simulink model "VIRTUAL_self_driving_stack_v2"  (R2024a)
settings: Solver=ode1  StartTime=0.0  StopTime=inf  FixedStep=Controller_Sample_Time  RelTol=1e-3  EnableMultiTasking=on
values from neighbouring files (symbols this model uses):
  angles_qcar2 = angles_new_qcar2(2: length (angles_new_qcar2), width (angles_new_qcar2)-5)    [Setup_QCar2_Params.m]
  cal_pos = [0, 0, 0]    [Setup_QCar2_Params.m]    (also in Setup_QCar2_Params_Addons.m)
  Controller_Sample_Time = 1/500    (= 0.002)    [Setup_QCar2_Params.m]    (also in Setup_QCar2_Params_Addons.m)
  CSI_Sample_Time = Controller_Sample_Time * ceil(0.033 / Controller_Sample_Time)    [Setup_QCar2_Params.m]
  GyroKF_P0 = eye(2)    [Setup_QCar2_Params.m]
  GyroKF_Q = diag([0.01, 0.001])    [Setup_QCar2_Params.m]
  GyroKF_R = 0.01    [Setup_QCar2_Params.m]
  GyroKF_X0 = [0;0]    [Setup_QCar2_Params.m]
  ImageDisplay_Sample_Time = Controller_Sample_Time * 50    (= 0.1)    [Setup_QCar2_Params.m]
  Initialization_Time = 5    [Setup_QCar2_Params.m]
  LiDAR_Sample_Time = Controller_Sample_Time * ceil(1/15 / Controller_Sample_Time)    [Setup_QCar2_Params.m]
  qcar2_lidar_to_body_rotation = -pi    (= -3.14159265359)    [Setup_QCar2_Params.m]
  qcar2_lidar_to_map_rotation = 0    [Setup_QCar2_Params.m]
  qcar2_virtual_to_physical_lidar_rotation = 0    [Setup_QCar2_Params.m]
  QCarEKF_L = 0.256    [Setup_QCar2_Params.m]
  QCarEKF_P0 = eye(3)    [Setup_QCar2_Params.m]
  QCarEKF_Q = diag([0.00001, 0.00001, 0.00001])    [Setup_QCar2_Params.m]
  QCarEKF_R_combined = diag([0.1, 0.1, 0.01])    [Setup_QCar2_Params.m]
  QCarEKF_R_heading = diag(0.1)    [Setup_QCar2_Params.m]
  QcarKF_X0 = [0; 0; 0]    [Setup_QCar2_Params.m]
  range_qcar2 = distance_new_qcar2(2: length (distance_new_qcar2), width (distance_new_qcar2)-5)    [Setup_QCar2_Params.m]
  RealSense_Sample_Time = Controller_Sample_Time * ceil(0.033 / Controller_Sample_Time)    [Setup_QCar2_Params.m]
undefined symbols (not defined in the file or in its folder): AAAF5050, gcbh, height, HIL, JPEG, K12, left, MC, path_x4, path_y4, Point, qc_get_step_size, top, video_display_show, width
libraries: quarc_library x42, simulink x3, simulink_extras x3
(part 1 of 2)
settings Model: SimulationMode=external  ExtModeTrigDuration=10000  Creator=PKaram  LastModifiedBy=mgilewicz
settings SolverCC: AlgebraicLoopSolver=TrustRegion  PositivePriorityOrder=on  AutoInsertRateTranBlk=on
settings DataIOCC: ReturnWorkspaceOutputs=off
settings DebuggingCC: ParameterPrecisionLossMsg=none  UnconnectedInputMsg=warning  UnconnectedOutputMsg=warning  UnconnectedLineMsg=warning  ArithmeticOperatorsInVariantConditions=warning
settings ModelReferenceCC: EnableRefExpFcnMdlSchedulingChecks=on
settings SFSimCC: SimUseLocalCustomCode=off  CustomCodeUndefinedFunction=UseInterfaceOnly
settings RTWCC: Description=QUARC Win64 Target Using Toolchain  SystemTargetFile=quarc_win64.tlc  TemplateMakefile=quarc_linux_nvidia_tmf  RTWUseLocalCustomCode=off  Toolchain=QUARC win64 | nmake (64-bit Windows)  BuildConfiguration=Faster Runs  GPUComputeCapability=3.5  DLArmComputeVersion=19.05
settings CodeAppCC: StateflowObjectComments=on
settings STFCustomTargetCC: ConcurrentExecutionCompliant=on  SystemTargetFile=quarc_win64.tlc
settings GRTTargetCC: ParMdlRefBuildCompliant=off  CompOptLevelCompliant=off  CombineOutputUpdateFcns=off  MatFileLogging=off  CPPClassGenCompliant=off  GRTInterface=on  ExtMode=on  ExtModeMexFile=quarc_comm
settings ConfigComp: CovMetricSettings=dswe  CovBoundaryAbsTol=1.0e-5

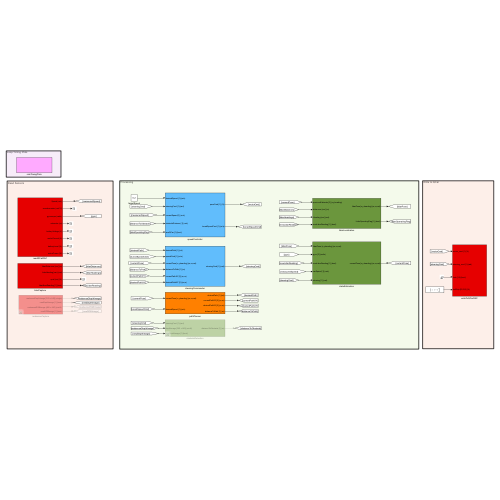
[thumbnail: Simulink's stored preview of the top-level diagram]
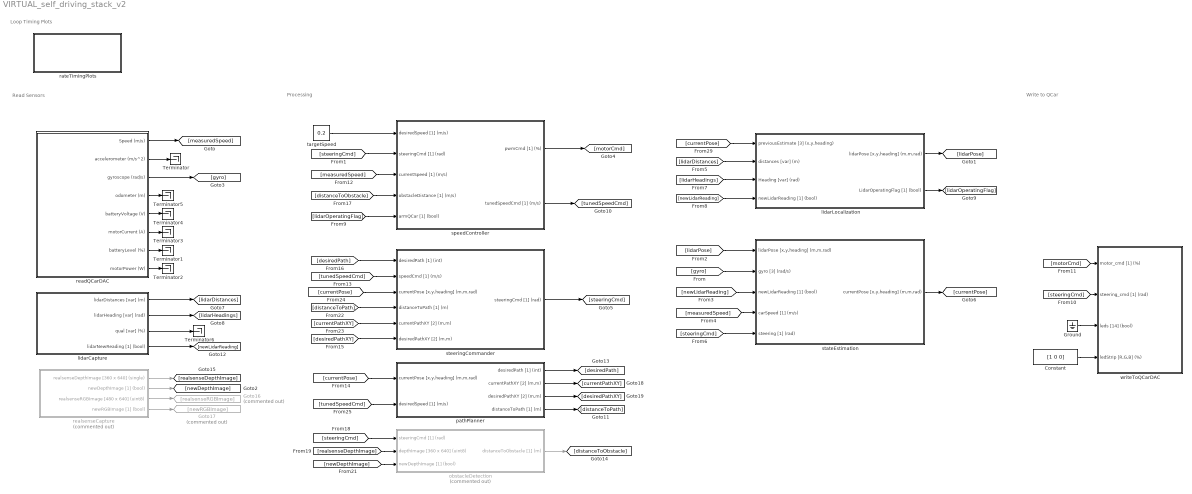
== system VIRTUAL_self_driving_stack_v2 ==
  note: Loop Timing Plots
  note: Write to QCar
  note: Processing
  note: Read Sensors
  Constant : Constant  Value=[1 0 0]
  Goto16 : Goto  Commented=on  GotoTag=realsenseRGBImage
  Goto17 : Goto  Commented=on  GotoTag=newRGBImage
  Ground : Ground
  Terminator{,1..6} (7 alike) : Terminator
  lidarCapture : Subsystem
  lidarLocalization : Subsystem
  obstacleDetection : Subsystem  Commented=on
  pathPlanner : Subsystem
  rateTimingPlots : Subsystem
  readQCarDAC : Subsystem
  realsenseCapture : Subsystem  Commented=on
  speedController : Subsystem
  stateEstimation : Subsystem
  steeringCommander : Subsystem
  targetSpeed : Constant  Value=0.2
  writeToQCarDAC : Subsystem
  wires:
  readQCarDAC/6(motorCurrent (A)) -> Terminator3/1
  [measuredSpeed] -> stateEstimation/4(carSpeed [1] (m/s))
  [newLidarReading] -> stateEstimation/3(newLidarReading [1] (bool))
  [tunedSpeedCmd] -> steeringCommander/2(speedCmd [1] (m/s))
  Constant/1 -> writeToQCarDAC/4(ledStrip [R,G,B] (%))
  pathPlanner/2(currentPathXY [2] (m,m)) -> [currentPathXY]
  lidarCapture/2(lidarHeading [var] (rad)) -> [lidarHeadings]
  readQCarDAC/2(accelerometer (m/s^2)) -> Terminator/1
  lidarLocalization/2(LidarOperatingFlag [1] (bool)) -> [lidarOperatingFlag]
  Ground/1 -> writeToQCarDAC/3(leds [14] (bool))
  [lidarHeadings] -> lidarLocalization/3(Heading [var] (rad))
  realsenseCapture/1(realsenseDepthImage [360 x 640] (single)) -> [realsenseDepthImage]
  [steeringCmd] -> writeToQCarDAC/2(steering_cmd [1] (rad))
  pathPlanner/4(distanceToPath [1] (m)) -> [distanceToPath]
  lidarCapture/1(lidarDistances [var] (m)) -> [lidarDistances]
  readQCarDAC/4(odometer (m)) -> Terminator5/1
  readQCarDAC/3(gyroscope (rad/s)) -> [gyro]
  pathPlanner/3(desiredPathXY [2] (m,m)) -> [desiredPathXY]
  [newLidarReading] -> lidarLocalization/4(newLidarReading [1] (bool))
  [newDepthImage] -> obstacleDetection/3(newDepthImage [1] (bool))
  [tunedSpeedCmd] -> pathPlanner/2(desiredSpeed [1] (m/s))
  readQCarDAC/5(batteryVoltage (V)) -> Terminator4/1
  readQCarDAC/1(Speed (m/s)) -> [measuredSpeed]
  speedController/2(tunedSpeedCmd [1] (m/s)) -> [tunedSpeedCmd]
  [distanceToObstacle] -> speedController/4(obstacleDistance [1] (m/s))
  [gyro] -> stateEstimation/2(gyro [3] (rad/s))
  [currentPathXY] -> steeringCommander/5(currentPathXY [2] (m,m))
  [lidarPose] -> stateEstimation/1(lidarPose [x,y,heading] (m,m,rad))
  targetSpeed/1 -> speedController/1(desiredSpeed [1] (m/s))
  [steeringCmd] -> stateEstimation/5(steering [1] (rad))
  [realsenseDepthImage] -> obstacleDetection/2(depthImage [360 x 640] (uint8))
  readQCarDAC/8(motorPower (W)) -> Terminator2/1
  speedController/1(pwmCmd [1] (%)) -> [motorCmd]
  [lidarDistances] -> lidarLocalization/2(distances [var] (m))
  [lidarOperatingFlag] -> speedController/5(armQCar [1] (bool))
  [motorCmd] -> writeToQCarDAC/1(motor_cmd [1] (%))
  [steeringCmd] -> speedController/2(steeringCmd [1] (rad))
  lidarCapture/4(lidarNewReading [1] (bool)) -> [newLidarReading]
  lidarLocalization/1(lidarPose [x,y,heading] (m,m,rad)) -> [lidarPose]
  [desiredPathXY] -> steeringCommander/6(desiredPathXY [2] (m,m))
  [distanceToPath] -> steeringCommander/4(distanceToPath [1] (m))
  realsenseCapture/4(newRGBImage [1] (bool)) -> Goto17/1
  lidarCapture/3(qual [var] (%)) -> Terminator6/1
  readQCarDAC/7(batteryLevel (%)) -> Terminator1/1
  [desiredPath] -> steeringCommander/1(desiredPath [1] (int))
  [steeringCmd] -> obstacleDetection/1(steeringCmd [1] (rad))
  steeringCommander/1(steeringCmd [1] (rad)) -> [steeringCmd]
  obstacleDetection/1(distanceToObstacle [1] (m)) -> [distanceToObstacle]
  [measuredSpeed] -> speedController/3(currentSpeed [1] (m/s))
  pathPlanner/1(desiredPath [1] (int)) -> [desiredPath]
  realsenseCapture/2(newDepthImage [1] (bool)) -> [newDepthImage]
  realsenseCapture/3("realsenseRGBImage [480 x 640] (uint8) ") -> Goto16/1
  stateEstimation/1(currentPose [x,y,heading] (m,m,rad)) -> [currentPose]
  [currentPose] -> pathPlanner/1(currentPose [x,y,heading] (m,m,rad))
  [currentPose] -> steeringCommander/3(currentPose [x,y,heading] (m,m,rad))
  [currentPose] -> lidarLocalization/1(previousEstimate [3] (x,y,heading))

== system VIRTUAL_self_driving_stack_v2/lidarCapture ==
  Ranging Sensor : quarc_library/Devices/Third-Party/Sensors/Ranging Sensor  sensor_type=RPLidar LIDAR  uri=tcpip://localhost:18966  ranging_distance=Long  timing_budget=0.033  measurement_period=0.040  output_mode=Variable-size output  samples_per_revolution=SPR_qcar2  max_distance=0.050  max_angle=5  sample_time=LiDAR_Sample_Time  show_versions=on  active=on
      settings: SourceProductName=QUARC Targets
  Terminator : Terminator
  lidarFirmwareVer : Display
      settings: Decimation=100
  lidarHardwareVer : Display
      settings: Decimation=100
  lidarModel : Display
      settings: Decimation=100
  virtualLidarToPhysicalLidarOffset : Bias  Bias=qcar2_virtual_to_physical_lidar_rotation  SaturateOnIntegerOverflow=off
  lidarDistances [var] (m) : Outport  VectorParamsAs1DForOutWhenUnconnected=off
  lidarHeading [var] (rad) : Outport  Port=2  VectorParamsAs1DForOutWhenUnconnected=off
  qual [var] (%) : Outport  Port=3  VectorParamsAs1DForOutWhenUnconnected=off
  lidarNewReading [1] (bool) : Outport  Port=4  VectorParamsAs1DForOutWhenUnconnected=off
  wires:
  Ranging Sensor/3 -> virtualLidarToPhysicalLidarOffset/1
  Ranging Sensor/5 -> lidarNewReading [1] (bool)/1
  Ranging Sensor/7 -> lidarHardwareVer/1
  Ranging Sensor/8 -> lidarFirmwareVer/1
  Ranging Sensor/6 -> lidarModel/1
  Ranging Sensor/4 -> qual [var] (%)/1
  Ranging Sensor/1 -> lidarDistances [var] (m)/1
  Ranging Sensor/2 -> Terminator/1
  virtualLidarToPhysicalLidarOffset/1 -> lidarHeading [var] (rad)/1

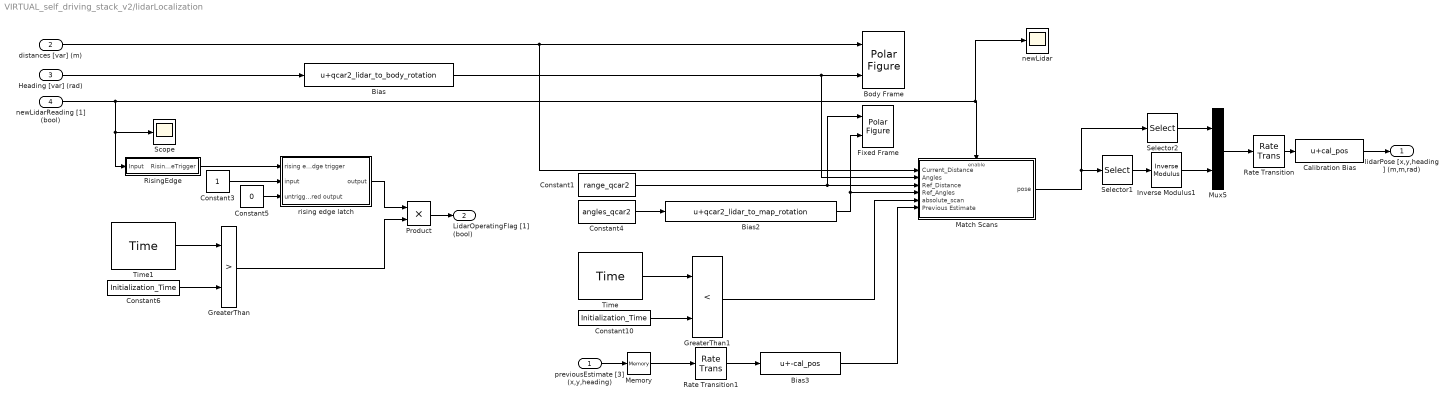
== system VIRTUAL_self_driving_stack_v2/lidarLocalization ==
  previousEstimate [3] (x,y,heading) : Inport
  distances [var] (m) : Inport  Port=2
  Heading [var] (rad) : Inport  Port=3
  newLidarReading [1] (bool) : Inport  Port=4
  Bias : Bias  Bias=qcar2_lidar_to_body_rotation  SaturateOnIntegerOverflow=off
  Bias2 : Bias  Bias=qcar2_lidar_to_map_rotation  SaturateOnIntegerOverflow=off
  Bias3 : Bias  Bias=-cal_pos  SaturateOnIntegerOverflow=off
  Body Frame : quarc_library/Sinks/Figures/Polar Figure  figure_mode=Use figure window  figure_tag=figure1  axes_tag=axes1  plot_mode=Frame-based  minimum_rho=0  maximum_rho=10  minimum_theta=0  maximum_theta=360  zero_location=top  direction=clockwise  buffer_size=SPR_qcar2  update_rate=1  sample_time=-1  initial_position="-958   50  958  973"  initial_visibility=off  line1_style=None  line1_width=0.5  line1_color=[0 0.4470 0.7410]  marker1=Point (.)  marker1_size=1  marker1_edge_color=[0 0.447059 0.741176]  marker1_face_color=[0 0.447059 0.741176]  line2_style=Solid line (-)  line2_width=0.5  line2_color=[0.85098 0.32549 0.0980392]  marker2=None  marker2_size=6  marker2_edge_color=[0.85098 0.32549 0.0980392]  marker2_face_color=[0.85098 0.32549 0.0980392]  line3_style=Solid line (-)  line3_width=0.5  line3_color=[0.929412 0.694118 0.12549]  marker3=None  marker3_size=6  marker3_edge_color=[0.929412 0.694118 0.12549]  marker3_face_color=[0.929412 0.694118 0.12549]  line4_style=Solid line (-)  line4_width=0.5  line4_color=[0.494118 0.184314 0.556863]  marker4=None  marker4_size=6  marker4_edge_color=[0.494118 0.184314 0.556863]  marker4_face_color=[0.494118 0.184314 0.556863]  line5_style=Solid line (-)  line5_width=0.5  line5_color=[0.466667 0.67451 0.188235]  marker5=None  marker5_size=6  marker5_edge_color=[0.466667 0.67451 0.188235]  marker5_face_color=[0.466667 0.67451 0.188235]
      settings: SourceProductName=QUARC Targets
  Calibration Bias : Bias  Bias=cal_pos  SaturateOnIntegerOverflow=off
  Constant1 : Constant  Value=range_qcar2
  Constant10 : Constant  Value=Initialization_Time
  Constant3 : Constant
  Constant4 : Constant  Value=angles_qcar2
  Constant5 : Constant  Value=0
  Constant6 : Constant  Value=Initialization_Time
  Fixed Frame : quarc_library/Sinks/Figures/Polar Figure  figure_mode=Use figure window  figure_tag=figure1  axes_tag=axes1  plot_mode=Frame-based  minimum_rho=0  maximum_rho=6  minimum_theta=0  maximum_theta=360  zero_location=top  direction=clockwise  buffer_size=SPR_qcar2  update_rate=1  sample_time=-1  initial_position="-1918    50   958   973"  initial_visibility=off  line1_style=None  line1_width=0.5  line1_color=[0 0.4470 0.7410]  marker1=Point (.)  marker1_size=1  marker1_edge_color=[0 0.447059 0.741176]  marker1_face_color=[0 0.447059 0.741176]  line2_style=Solid line (-)  line2_width=0.5  line2_color=[0.85098 0.32549 0.0980392]  marker2=None  marker2_size=6  marker2_edge_color=[0.85098 0.32549 0.0980392]  marker2_face_color=[0.85098 0.32549 0.0980392]  line3_style=Solid line (-)  line3_width=0.5  line3_color=[0.929412 0.694118 0.12549]  marker3=None  marker3_size=6  marker3_edge_color=[0.929412 0.694118 0.12549]  marker3_face_color=[0.929412 0.694118 0.12549]  line4_style=Solid line (-)  line4_width=0.5  line4_color=[0.494118 0.184314 0.556863]  marker4=None  marker4_size=6  marker4_edge_color=[0.494118 0.184314 0.556863]  marker4_face_color=[0.494118 0.184314 0.556863]  line5_style=Solid line (-)  line5_width=0.5  line5_color=[0.466667 0.67451 0.188235]  marker5=None  marker5_size=6  marker5_edge_color=[0.466667 0.67451 0.188235]  marker5_face_color=[0.466667 0.67451 0.188235]
      settings: SourceProductName=QUARC Targets
  GreaterThan : RelationalOperator  Operator=>  OutDataTypeStr=boolean  RndMeth=Simplest  InputSameDT=off
  GreaterThan1 : RelationalOperator  Operator=<  OutDataTypeStr=boolean  RndMeth=Simplest  InputSameDT=off
  Inverse Modulus1 : quarc_library/Discontinuities/Inverse Modulus  modulus=2*pi  output_derivative=off  output_revolutions=off  max_x=Inf  min_x=-Inf
  Match Scans : Subsystem
  Memory : Memory
  Mux5 : Mux  Inputs=2
  Product : Product
  Rate Transition : RateTransition
  Rate Transition1 : RateTransition
  RisingEdge : Subsystem
  Scope : Scope
  Selector1 : Selector  InputPortWidth=3  IndexOptions=Index vector (dialog)  Indices=3  OutputSizes=1
  Selector2 : Selector  InputPortWidth=3  IndexOptions=Index vector (dialog)  Indices=1:2  OutputSizes=1
  Time : quarc_library/Sources/Time/Time  time_source=Wall clock  sample_time=LiDAR_Sample_Time
  Time1 : quarc_library/Sources/Time/Time  time_source=Wall clock  sample_time=qc_get_step_size
  newLidar : Scope
  rising edge latch : Subsystem
  lidarPose [x,y,heading] (m,m,rad) : Outport
  LidarOperatingFlag [1] (bool) : Outport  Port=2
  wires:
  RisingEdge/1(RisingEdgeTrigger) -> rising edge latch/1(rising edge trigger)
  Bias3/1 -> Match Scans/6(Previous Estimate)
  Inverse Modulus1/1 -> Mux5/2
  Constant1/1 -> Fixed Frame/1, Match Scans/3(Ref_Distance)
  Time1/1 -> GreaterThan/1
  Rate Transition1/1 -> Bias3/1
  Bias2/1 -> Fixed Frame/2, Match Scans/4(Ref_Angles)
  Constant3/1 -> rising edge latch/2(input)
  GreaterThan/1 -> Product/2
  Selector2/1 -> Mux5/1
  Bias/1 -> Body Frame/2, Match Scans/2(Angles)
  Constant10/1 -> GreaterThan1/2
  Mux5/1 -> Rate Transition/1
  rising edge latch/1(output) -> Product/1
  Constant6/1 -> GreaterThan/2
  Heading [var] (rad)/1 -> Bias/1
  distances [var] (m)/1 -> Match Scans/1(Current_Distance), Body Frame/1
  Time/1 -> GreaterThan1/1
  Match Scans/1(pose) -> Selector2/1, Selector1/1
  Product/1 -> LidarOperatingFlag [1] (bool)/1
  Constant4/1 -> Bias2/1
  newLidarReading [1] (bool)/1 -> newLidar/1, Match Scans/Enable, RisingEdge/1(Input), Scope/1
  GreaterThan1/1 -> Match Scans/5(absolute_scan)
  Selector1/1 -> Inverse Modulus1/1
  Calibration Bias/1 -> lidarPose [x,y,heading] (m,m,rad)/1
  previousEstimate [3] (x,y,heading)/1 -> Memory/1
  Rate Transition/1 -> Calibration Bias/1
  Constant5/1 -> rising edge latch/3(untriggered output)
  Memory/1 -> Rate Transition1/1

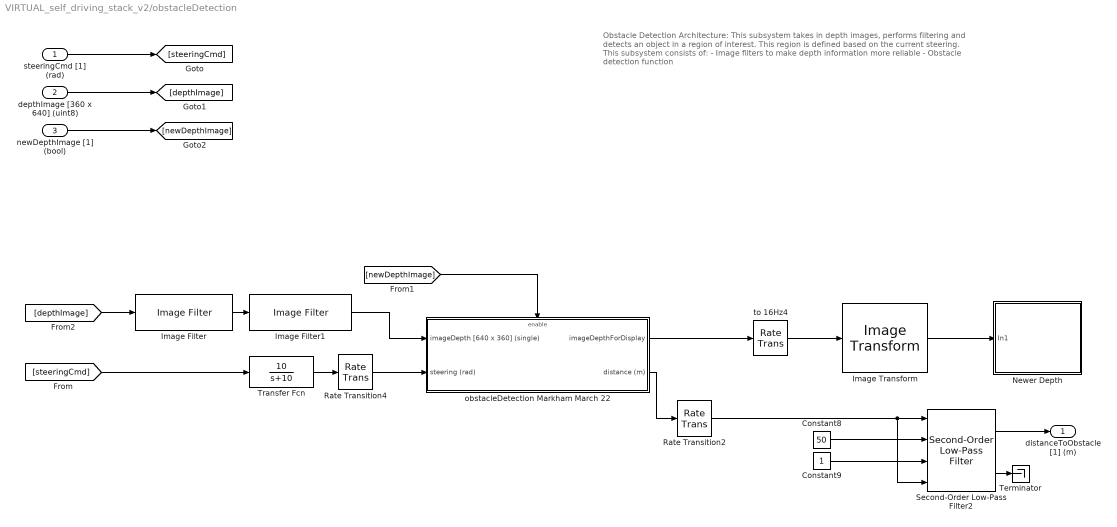
== system VIRTUAL_self_driving_stack_v2/obstacleDetection ==
  note: Obstacle Detection Architecture:
      |
      | This subsystem takes in depth images, performs filtering and detects an object in a region of interest. This region is defined based on the current steering.
      |
      | This subsystem consists of:
      |
      | - Image filters to make depth information more reliable
      | - Obstacle detection function
  steeringCmd [1] (rad) : Inport
  depthImage [360 x 640] (uint8) : Inport  Port=2
  newDepthImage [1] (bool) : Inport  Port=3
  Constant8 : Constant  Value=50
  Constant9 : Constant
  Image Filter : quarc_library/Image Processing/Generic/Image Filter  filter_type=Depth hole-fill  source_of_roi=Internal dialog parameter  roi_style=[top, left, height, width]  roi=[]  maximum_roi=[]  roi_zone=Operate inside region of interest  border_type=Replicate  border_value=[0 0 0]  kernel_size=5  sigma=10  mask_size=[3 3]  kernel=int16([-2 -1 0; -1 1 1; 0 1 2])  divisor=1  offset=0  rounding=Nearest  algorithm_hint=None  threshold=100  alpha=0.9  num_frames=8  num_valid=1  gap_threshold=10  depth_threshold=255  iterations=2  norm_type=L1
      settings: AttributesFormatString=(%<filter_type>)  SourceProductName=QUARC Targets
  Image Filter1 : quarc_library/Image Processing/Generic/Image Filter  filter_type=Depth temporal low-pass  source_of_roi=Internal dialog parameter  roi_style=[top, left, height, width]  roi=[]  maximum_roi=[]  roi_zone=Operate inside region of interest  border_type=Replicate  border_value=[0 0 0]  kernel_size=5  sigma=10  mask_size=[3 3]  kernel=int16([-2 -1 0; -1 1 1; 0 1 2])  divisor=1  offset=0  rounding=Nearest  algorithm_hint=None  threshold=100  alpha=0.9  num_frames=4  num_valid=1  gap_threshold=10  depth_threshold=255  iterations=2  norm_type=L1
      settings: AttributesFormatString=(%<filter_type>)  SourceProductName=QUARC Targets
  Image Transform : quarc_library/Image Processing/Generic/Image Transform  algorithm=Colorize  color_theme=KRYGCBMW  min_pixel=0  max_pixel=65535  contour_depth=1  focal_length=308  principal_point=[262 334]  radial_coeffs=[-0.3129 0.0907]  tangential_coeffs=[]  extrapolated_pixel=0  interpolation=nearest  row_coords=0  column_coords=0  output_height=480  output_width=640  angle=0  origin=[240 320]  output_origin=[240 320]  output_data_type=uint8
      settings: AttributesFormatString=(%<algorithm>)  SourceProductName=QUARC Targets
  Newer Depth : Subsystem  LoadFcn=set_param(gcbh, 'UserData', gcb);  StartFcn=video_display_show([gcb, '/Video Display'], 'add', gcb);  mask(Video Compressed Display){algorithm=JPEG, quality=50, sample_time=-1, use_hardware=on}
      mask prompts: algorithm "Compression algorithm:"; quality "Compression quality (0-100):"; sample_time "Sample time (seconds):"; use_hardware "Use hardware acceleration for video display"
      mask help: Displays a video stream on the host, using compression to minimize bandwidth.
      mask init:
      | qc_set_display('Video\nCompressed\nDisplay');
      settings: UndoDeleteFcn=set_param(gcbh, 'UserData', gcb);  OpenFcn=video_display_show([gcb, '/Video Display'], 'show', gcb);  PreDeleteFcn=video_display_show([gcb, '/Video Display'], 'delete');
      settings: CopyFcn=|
      | set_param(gcbh, 'UserData', gcb);
      | set_param(gcbh, 'LinkStatus', 'none');
      settings: NameChangeFcn=|
      | video_display_show([get_param(gcbh, 'UserData'), '/Video Display'], 'rename', [gcb, '/Video Display']);
      | video_display_show([gcb, '/Video Display'], 'add', gcb);
      | set_param(gcbh, 'UserData', gcb);
      mask Help: web(qc_get_block_help_path(gcb));
      mask TypeOptions algorithm: Image Compress/algorithm
      mask TypeOptions quality: Image Compress/quality
      mask TypeOptions sample_time: Video Display/sample_time
      mask TypeOptions use_hardware: Video Display/use_hardware
      mask Display:
      | patch([0.98591 0.98591 0.62618 0.59072 0.56147   0.536   0.536  0.5441 0.56912 0.59207 0.60881 0.62276 0.63527 0.64364  0.6485  0.6485 0.64706 0.64499 0.63662 0.62411 0.61232 0.59837 0.58307 0.56147   0.536   0.536  0.5441  0.5747 0.60953 0.63662 0.67001  0.7034 0.72851 0.75425 0.77927 0.80294 0.82454 0.84119 0.85865 0.87395 0.88574 0.89339  0.8969 0.89969 0.89969 0.89267  0.8816 0.87044 0.85649  0.8384 0.81824 0.80294 0.78764 0.77513 0.76676 0.75776 0.76397 0.77513 0.79178 0.80987 0.82796 0.84326 0.86207 0.98528],[0.18689 0.05522 0.05522 0.05171 0.05171    0.05 0.18338 0.18338 0.19148 0.20435 0.22298 0.24863 0.28589 0.33125 0.38138 0.55139 0.59801 0.63761 0.68189 0.72149 0.74939 0.76694 0.77855 0.79367 0.79952 0.92768 0.92768 0.92768 0.92417 0.92066 0.91364  0.9032 0.89384 0.88106 0.86594 0.85073 0.82634 0.80537 0.77855 0.74363 0.70403 0.65858 0.61079 0.59099 0.41513 0.37202 0.31847 0.29048 0.25556 0.23342  0.2102 0.19382 0.18221 0.17285 0.16943 0.16124  0.1589 0.16241 0.16709 0.17168  0.1787 0.18221 0.18689 0.18689],[0.9,0.90,0.91])
      | patch([0.536 0.52601 0.46823 0.44528 0.41603 0.39101 0.35555 0.33116 0.31451 0.29291  0.2804 0.26717 0.25322 0.23999 0.22406 0.20732 0.19337 0.17528 0.15935 0.14396 0.13217 0.11759 0.10922 0.10085 0.09671 0.09392 0.09041 0.08906 0.08906 0.09464  0.0995 0.10778 0.11894 0.13145 0.14675 0.16349 0.17672 0.19409 0.20732 0.22406 0.23999 0.26159 0.27833 0.29849 0.31793 0.33602 0.35411 0.37085 0.39245 0.41603   0.536   0.536 0.53159 0.46409   0.446 0.42026 0.39587 0.37571 0.36113 0.34925 0.34088 0.33809 0.33809 0.34088 0.34583 0.35627 0.36392 0.38129 0.39587 0.41117 0.42719 0.44672  0.4676 0.48353 0.48353 0.52394   0.536],[0.05 0.04829 0.04712 0.04712 0.04829 0.05063 0.05405 0.05873 0.06107 0.06692 0.07043 0.07619 0.08087 0.08672 0.09482 0.10652 0.11696 0.13325  0.1508 0.17168 0.19499 0.22415 0.25439 0.28472 0.31379 0.35456 0.38489 0.41513 0.58055 0.63878 0.68774 0.72149 0.75641 0.78089 0.80537 0.82859 0.84029 0.85658 0.86594 0.87404  0.8834 0.89267 0.90086 0.90788 0.91247 0.91832 0.92066   0.923 0.92651 0.92768 0.92768 0.79952 0.79952 0.79952 0.79718 0.78899 0.77153 0.75056 0.72149 0.68072 0.62249  0.5549 0.41396 0.37085 0.33242 0.28121 0.25205 0.22181 0.20552 0.19499 0.18572 0.18221 0.17753 0.17636 0.17753  0.1787  0.1787],[0.9,0.90,0.91])
      | disp('Video\nCompressed\nDisplay');
  Rate Transition2 : RateTransition
  Rate Transition4 : RateTransition
  Second-Order Low-Pass Filter2 : quarc_library/Continuous/Second-Order Low-Pass Filter  params_source=External (input ports)  input_width=1  input_zeta=1  input_init=0
  Terminator : Terminator
  Transfer Fcn : TransferFcn  Numerator=[10]  Denominator=[1 10]
  obstacleDetection Markham March 22 : Subsystem
  to 16Hz4 : RateTransition  OutPortSampleTime=ImageDisplay_Sample_Time
  distanceToObstacle [1] (m) : Outport
  wires:
  Transfer Fcn/1 -> Rate Transition4/1
  steeringCmd [1] (rad)/1 -> [steeringCmd]
  Constant9/1 -> Second-Order Low-Pass Filter2/3
  obstacleDetection Markham March 22/2(distance (m)) -> Rate Transition2/1
  Rate Transition2/1 -> Second-Order Low-Pass Filter2/4, Second-Order Low-Pass Filter2/1
  obstacleDetection Markham March 22/1(imageDepthForDisplay) -> to 16Hz4/1
  Second-Order Low-Pass Filter2/2 -> Terminator/1
  Rate Transition4/1 -> obstacleDetection Markham March 22/2(steering (rad))
  Constant8/1 -> Second-Order Low-Pass Filter2/2
  Second-Order Low-Pass Filter2/1 -> distanceToObstacle [1] (m)/1
  to 16Hz4/1 -> Image Transform/1
  Image Transform/1 -> Newer Depth/1(In1)
  [steeringCmd] -> Transfer Fcn/1
  Image Filter/1 -> Image Filter1/1
  depthImage [360 x 640] (uint8)/1 -> [depthImage]
  newDepthImage [1] (bool)/1 -> [newDepthImage]
  [newDepthImage] -> obstacleDetection Markham March 22/Enable
  [depthImage] -> Image Filter/1
  Image Filter1/1 -> obstacleDetection Markham March 22/1(imageDepth [640 x 360] (single))

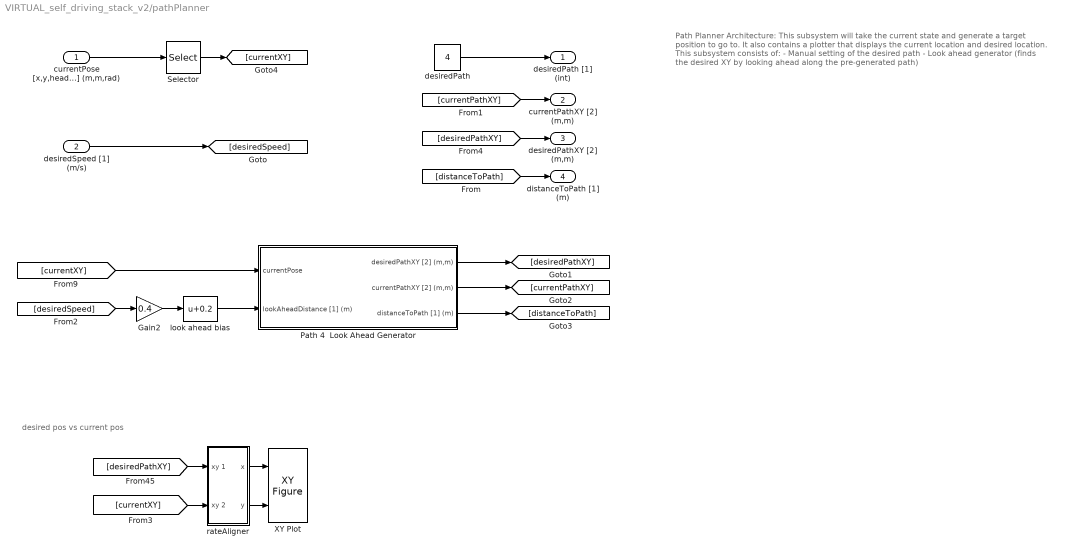
== system VIRTUAL_self_driving_stack_v2/pathPlanner ==
  note: desired pos vs current pos
  note: Path Planner Architecture:
      |
      | This subsystem will take the current state and generate a target position to go to. It also contains a plotter that displays the current location and desired location.
      |
      | This subsystem consists of:
      |
      | - Manual setting of the desired path
      | - Look ahead generator (finds the desired XY by looking ahead along the pre-generated path)
  currentPose [x,y,heading] (m,m,rad) : Inport
  desiredSpeed [1] (m/s) : Inport  Port=2
  Gain2 : Gain  Gain=0.4
  Path 4  Look Ahead Generator : Subsystem
  Selector : Selector  InputPortWidth=3  IndexOptions=Index vector (dialog)  Indices=[1 2]  OutputSizes=1
  XY Plot : quarc_library/Sinks/Figures/XY Figure  figure_mode=Use figure window  figure_tag=figure1  axes_tag=axes1  plot_mode=Time-based  minimum_x=-2.5  maximum_x=2.5  minimum_y=-2  maximum_y=5  buffer_size=100  update_rate=1  initial_position="-958   50  958  973"  initial_visibility=off  sample_time=-1
      settings: SourceProductName=QUARC Targets
  desiredPath : Constant  Value=4
  look ahead bias : Bias  Bias=0.2  SaturateOnIntegerOverflow=off
  rateAligner : Subsystem
  desiredPath [1] (int) : Outport
  currentPathXY [2] (m,m) : Outport  Port=2
  desiredPathXY [2] (m,m) : Outport  Port=3
  distanceToPath [1] (m) : Outport  Port=4
  wires:
  desiredPath/1 -> desiredPath [1] (int)/1
  [desiredSpeed] -> Gain2/1
  Gain2/1 -> look ahead bias/1
  [currentXY] -> Path 4  Look Ahead Generator/1(currentPose)
  look ahead bias/1 -> Path 4  Look Ahead Generator/2(lookAheadDistance [1] (m))
  rateAligner/1(x) -> XY Plot/1
  rateAligner/2(y) -> XY Plot/2
  [desiredPathXY] -> rateAligner/1(xy 1)
  [currentXY] -> rateAligner/2(xy 2)
  currentPose [x,y,heading] (m,m,rad)/1 -> Selector/1
  desiredSpeed [1] (m/s)/1 -> [desiredSpeed]
  Path 4  Look Ahead Generator/1(desiredPathXY [2] (m,m)) -> [desiredPathXY]
  Selector/1 -> [currentXY]
  Path 4  Look Ahead Generator/2(currentPathXY [2] (m,m)) -> [currentPathXY]
  Path 4  Look Ahead Generator/3(distanceToPath [1] (m)) -> [distanceToPath]
  [distanceToPath] -> distanceToPath [1] (m)/1
  [currentPathXY] -> currentPathXY [2] (m,m)/1
  [desiredPathXY] -> desiredPathXY [2] (m,m)/1

== system VIRTUAL_self_driving_stack_v2/rateTimingPlots ==
  CSI : Scope
  Control : Scope
  Image Displays : Scope
  LCD : Scope
  LiDAR : Scope
  RealSense : Scope
  monitorTiming : Subsystem
  monitorTiming1 : Subsystem
  monitorTiming2 : Subsystem
  monitorTiming3 : Subsystem
  monitorTiming5 : Subsystem
  monitorTiming7 : Subsystem
  wires:
  monitorTiming/1(Timing (s)) -> CSI/1
  monitorTiming1/1(Timing (s)) -> Control/1
  monitorTiming3/1(Timing (s)) -> Image Displays/1
  monitorTiming2/1(Timing (s)) -> RealSense/1
  monitorTiming5/1(Timing (s)) -> LiDAR/1
  monitorTiming7/1(Timing (s)) -> LCD/1

== system VIRTUAL_self_driving_stack_v2/readQCarDAC ==
  HIL Initialize : quarc_library/Data Acquisition/Generic/Configuration/HIL Initialize  object_name=HIL-2  board_type=qcar2  board_number=0@tcpip://localhost:18960  board_options=gyro_fs=250;gyro_rate=500;gyro_bw=125;gyro_ord=3;accel_fs=4;accel_rate=500;accel_bw=250;accel_ord=3;temp_bw=4000;enc0_dir=0;enc1_dir=0;enc2_dir=0;steer_bias=0.05;  exclusive=off  active=on  hardware_clocks=[]  clock_modes=[]  initial_clock_frequencies=[]  set_clock_params_at_start=off  set_clock_params_at_switch_in=off  set_clock_frequencies_at_start=off  set_clock_frequencies_at_switch_in=off  analog_input_channels=[0:4]  analog_input_configurations=[]  analog_input_maximums=[3.3]  analog_input_minimums=[0]  set_analog_input_params_at_start=off  set_analog_input_params_at_switch_in=off  analog_output_channels=[]  analog_output_maximums=[]  analog_output_minimums=[]  initial_analog_outputs=[]  final_analog_outputs=[]  watchdog_analog_outputs=[]  set_analog_output_params_at_start=off  set_analog_output_params_at_switch_in=off  set_analog_outputs_at_start=off  set_analog_outputs_at_switch_in=off  set_analog_outputs_at_terminate=off  set_analog_outputs_at_switch_out=off  set_analog_outputs_on_watchdog=off  digital_input_channels=[0:14]  digital_output_channels=[11:26]  digital_output_configuration=[]  initial_digital_outputs=[0]  final_digital_outputs=[0]  watchdog_digital_outputs=[0]  set_digital_output_params_at_start=off  set_digital_output_params_at_switch_in=off  set_digital_outputs_at_start=on  set_digital_outputs_at_switch_in=off  set_digital_outputs_at_terminate=on  set_digital_outputs_at_switch_out=off  set_digital_outputs_on_watchdog=off  encoder_channels=[0:2]  quadrature=[4]  encoder_filter_frequency=100e6/1  initial_encoder_counts=[0]  set_encoder_params_at_start=on  set_encoder_params_at_switch_in=off  set_encoder_counts_at_start=on  set_encoder_counts_at_switch_in=off  pwm_channels=[0:1]  pwm_modes=[0]  pwm_frequency=180e6/4096  pwm_configuration=[0]  pwm_alignment=[0]  pwm_polarity=[1]  pwm_leading_deadband=[]  pwm_trailing_deadband=[]  initial_pwm_outputs=[0]  final_pwm_outputs=[0]  watchdog_pwm_outputs=[0]  set_pwm_params_at_start=on  set_pwm_params_at_switch_in=off  set_pwm_outputs_at_start=on  set_pwm_outputs_at_switch_in=off  set_pwm_outputs_at_terminate=on  set_pwm_outputs_at_switch_out=off  set_pwm_outputs_on_watchdog=off  other_output_channels=[1000 11000]  initial_other_outputs=[0]  final_other_outputs=[0]  watchdog_other_outputs=[0]  set_other_outputs_at_start=on  set_other_outputs_at_switch_in=off  set_other_outputs_at_terminate=on  set_other_outputs_at_switch_out=off  set_other_outputs_on_watchdog=off
  HIL Read Timebase : quarc_library/Data Acquisition/Generic/Timebases/HIL Read Timebase  object_name=HIL-2  clock=0  analog_channels=[4 2]  encoder_channels=[0]  digital_channels=[]  other_channels=[3000:3002 4000:4002 14000]  active=on  vector_output=off  data_type_mode=Inherit via back propagation  encoder_data_type=double  digital_data_type=boolean  overflow_mode=Synchronize (for simulated cards only)  samples_in_buffer=max(ceil(1/qc_get_step_size), 1)
  Mux1 : Mux  Inputs=3
  Mux2 : Mux  Inputs=3
  Unwrap 2^24 : quarc_library/Discontinuities/Inverse Modulus  modulus=16777215  output_derivative=off  output_revolutions=off  max_x=Inf  min_x=-Inf
  counts to meters : Subsystem
  counts/s to m/s : Subsystem
  powerConsumptionMonitor : Subsystem
  Speed (m/s) : Outport  VectorParamsAs1DForOutWhenUnconnected=off
  accelerometer (m/s^2) : Outport  Port=2  VectorParamsAs1DForOutWhenUnconnected=off
  gyroscope (rad/s) : Outport  Port=3  VectorParamsAs1DForOutWhenUnconnected=off
  odometer (m) : Outport  Port=4  VectorParamsAs1DForOutWhenUnconnected=off
  batteryVoltage (V) : Outport  Port=5
  motorCurrent (A) : Outport  Port=6
  batteryLevel (%) : Outport  Port=7
  motorPower (W) : Outport  Port=8
  wires:
  HIL Read Timebase/3 -> Unwrap 2^24/1  "encoder counts"
  HIL Read Timebase/1 -> powerConsumptionMonitor/1(motorCurrent (A) [1]), motorCurrent (A)/1  "motor current"
  HIL Read Timebase/2 -> batteryVoltage (V)/1, powerConsumptionMonitor/2(batteryVoltage (V) [1])  "battery voltage"
  HIL Read Timebase/10 -> counts/s to m/s/1(motorSpeed (counts/s))
  Unwrap 2^24/1 -> counts to meters/1(motorSpeed (counts/s))
  counts to meters/1(longitudinalCarSpeed (m/s)) -> odometer (m)/1
  counts/s to m/s/1(longitudinalCarSpeed (m/s)) -> Speed (m/s)/1
  powerConsumptionMonitor/1(motorPowerConsumption (W) [1]) -> motorPower (W)/1
  powerConsumptionMonitor/2(batteryLevel (%) [1]) -> batteryLevel (%)/1
  HIL Read Timebase/4 -> Mux1/1  "x"
  HIL Read Timebase/5 -> Mux1/2  "y"
  HIL Read Timebase/6 -> Mux1/3  "z"
  Mux1/1 -> gyroscope (rad/s)/1
  HIL Read Timebase/7 -> Mux2/1  "x"
  HIL Read Timebase/8 -> Mux2/2  "y"
  HIL Read Timebase/9 -> Mux2/3  "z"
  Mux2/1 -> accelerometer (m/s^2)/1

== system VIRTUAL_self_driving_stack_v2/realsenseCapture ==
  Terminator : Terminator
  Terminator1 : Terminator  Commented=on
  Terminator2 : Terminator  Commented=on
  Terminator3 : Terminator
  Terminator4 : Terminator
  Video3D Initialize : quarc_library/Multimedia/Video3D Initialize  object_name=RealSense  source=Device  identifier=0@tcpip://localhost:18965  file=sample.bag  sample_time=RealSense_Sample_Time  active=on
  realsenseDepthCapture : quarc_library/Multimedia/Video3D Capture  object_name=unassigned  stream_type=Depth  stream_index=0  resolution=640 x 360  width=640  height=360  output_format=Distance in meters (HxW)  data_type=single  sample_time=RealSense_Sample_Time  camera_intrinsics=off  depth_scale=off  brightness_override=Do not override  brightness=50.0  contrast_override=Do not override  contrast=50.0  hue_override=Do not override  hue=50.0  saturation_override=Do not override  saturation=50.0  sharpness_override=Do not override  sharpness=50.0  gamma_override=Do not override  gamma=50.0  gain_override=Do not override  gain=50.0  backlightcompensation_override=Do not override  backlightcompensation=50.0  whitebalance_override=Automatic white balance  whitebalance=50.0  exposure_override=Automatic exposure  exposure=30.0  emitter=Enable laser emitter  preset=Do not set camera presets
  realsenseRGBCapture : quarc_library/Multimedia/Video3D Capture  Commented=on  object_name=unassigned  stream_type=RGB  stream_index=0  resolution=640 x 480  width=640  height=480  output_format=MATLAB RGB (HxWx3)  data_type=uint8  sample_time=RealSense_Sample_Time*1  camera_intrinsics=off  depth_scale=off  brightness_override=Do not override  brightness=50.0  contrast_override=Do not override  contrast=50.0  hue_override=Do not override  hue=50.0  saturation_override=Do not override  saturation=50.0  sharpness_override=Do not override  sharpness=50.0  gamma_override=Do not override  gamma=50.0  gain_override=Do not override  gain=50.0  backlightcompensation_override=Do not override  backlightcompensation=50.0  whitebalance_override=Automatic white balance  whitebalance=50.0  exposure_override=Automatic exposure  exposure=30.0  emitter=Enable laser emitter  preset=Do not set camera presets
  realsenseDepthImage [360 x 640] (single) : Outport
  newDepthImage [1] (bool) : Outport  Port=2
  "realsenseRGBImage [480 x 640] (uint8) " : Outport  Port=3
  newRGBImage [1] (bool) : Outport  Port=4
  wires:
  realsenseDepthCapture/4 -> newDepthImage [1] (bool)/1
  realsenseDepthCapture/2 -> Terminator4/1
  realsenseDepthCapture/3 -> Terminator3/1
  Video3D Initialize/1 -> Terminator/1
  realsenseRGBCapture/2 -> Terminator1/1
  realsenseRGBCapture/3 -> Terminator2/1
  realsenseDepthCapture/1 -> realsenseDepthImage [360 x 640] (single)/1
  realsenseRGBCapture/4 -> newRGBImage [1] (bool)/1
  realsenseRGBCapture/1 -> "realsenseRGBImage [480 x 640] (uint8) "/1

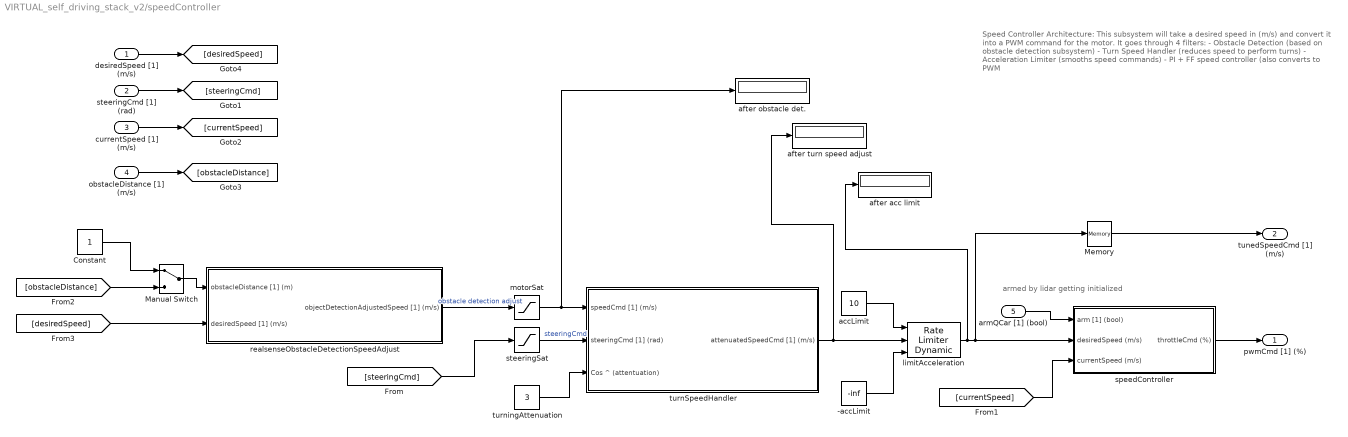
== system VIRTUAL_self_driving_stack_v2/speedController ==
  note: Speed Controller Architecture:
      |
      | This subsystem will take a desired speed in (m/s) and convert it into a PWM command for the motor.
      |
      | It goes through 4 filters:
      | - Obstacle Detection (based on obstacle detection subsystem)
      | - Turn Speed Handler (reduces speed to perform turns)
      | - Acceleration Limiter (smooths speed commands)
      | - PI + FF speed controller (also converts to PWM
  note: armed by lidar getting initialized
  desiredSpeed [1] (m/s) : Inport
  steeringCmd [1] (rad) : Inport  Port=2
  currentSpeed [1] (m/s) : Inport  Port=3
  obstacleDistance [1] (m/s) : Inport  Port=4
  armQCar [1] (bool) : Inport  Port=5
  -accLimit : Constant  Value=-inf
  Constant : Constant
  Manual Switch : ManualSwitch
  Memory : Memory
  accLimit : Constant  Value=10
  after acc limit : Display
  after obstacle det. : Display
  after turn speed adjust : Display
  limitAcceleration : simulink/Discontinuities/Rate Limiter Dynamic
  motorSat : Saturate  UpperLimit=3  LowerLimit=-3
  realsenseObstacleDetectionSpeedAdjust : Subsystem
  speedController : Subsystem
  steeringSat : Saturate  UpperLimit=0.6  LowerLimit=-0.6
  turnSpeedHandler : Subsystem
  turningAttenuation : Constant  Value=3
  pwmCmd [1] (%) : Outport
  tunedSpeedCmd [1] (m/s) : Outport  Port=2
  wires:
  steeringSat/1 -> turnSpeedHandler/2(steeringCmd [1] (rad))  "steeringCmd"
  speedController/1(throttleCmd (%)) -> pwmCmd [1] (%)/1
  armQCar [1] (bool)/1 -> speedController/1(arm [1] (bool))
  turningAttenuation/1 -> turnSpeedHandler/3(Cos ^ (attentuation))
  motorSat/1 -> after obstacle det./1, turnSpeedHandler/1(speedCmd [1] (m/s))
  turnSpeedHandler/1(attenuatedSpeedCmd [1] (m/s)) -> after turn speed adjust/1, limitAcceleration/2
  accLimit/1 -> limitAcceleration/1
  limitAcceleration/1 -> after acc limit/1, Memory/1, speedController/2(desiredSpeed (m/s))
  -accLimit/1 -> limitAcceleration/3
  Memory/1 -> tunedSpeedCmd [1] (m/s)/1
  steeringCmd [1] (rad)/1 -> [steeringCmd]
  currentSpeed [1] (m/s)/1 -> [currentSpeed]
  [steeringCmd] -> steeringSat/1
  obstacleDistance [1] (m/s)/1 -> [obstacleDistance]
  [currentSpeed] -> speedController/3(currentSpeed (m/s))
  desiredSpeed [1] (m/s)/1 -> [desiredSpeed]
  [desiredSpeed] -> realsenseObstacleDetectionSpeedAdjust/2(desiredSpeed [1] (m/s))
  realsenseObstacleDetectionSpeedAdjust/1(objectDetectionAdjustedSpeed [1] (m/s)) -> motorSat/1  "obstacle detection adjust"
  [obstacleDistance] -> Manual Switch/2
  Constant/1 -> Manual Switch/1
  Manual Switch/1 -> realsenseObstacleDetectionSpeedAdjust/1(obstacleDistance [1] (m))

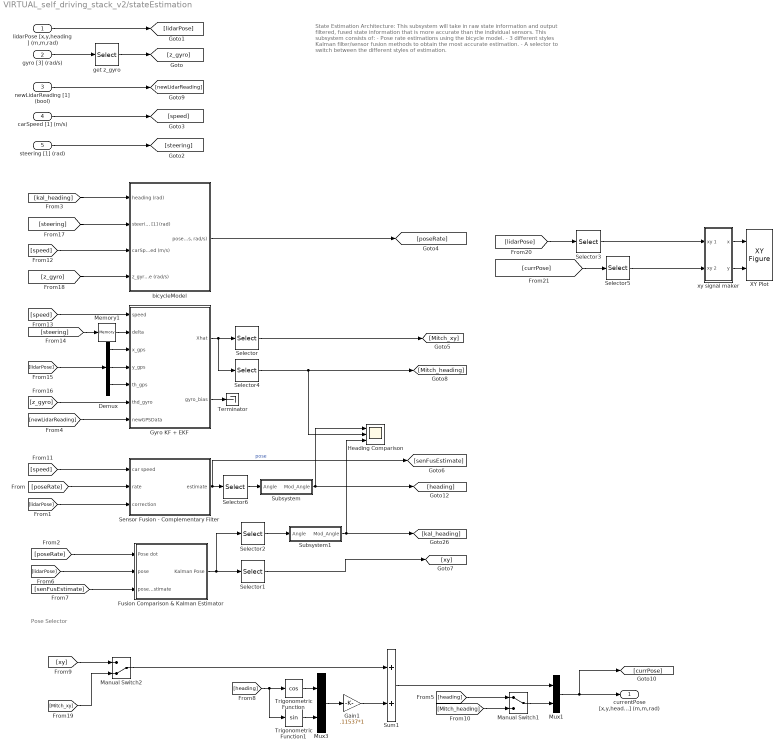
== system VIRTUAL_self_driving_stack_v2/stateEstimation ==
  note: Pose Selector
  note: State Estimation Architecture:
      |
      | This subsystem will take in raw state information and output filtered, fused state information that is more accurate than the individual sensors.
      |
      | This subsystem consists of:
      |
      | - Pose rate estimations using the bicycle model.
      | - 3 different styles Kalman filter/sensor fusion methods to obtain the most accurate estimation.
      | - A selector to switch between the different styles of estimation.
  lidarPose [x,y,heading] (m,m,rad) : Inport
  gyro [3] (rad/s) : Inport  Port=2
  newLidarReading [1] (bool) : Inport  Port=3
  carSpeed [1] (m/s) : Inport  Port=4
  steering [1] (rad) : Inport  Port=5
  Demux : Demux  Outputs=3
  Fusion Comparison & Kalman Estimator : Subsystem
  Gain1 : Gain  Gain=.11537*1
  Gyro KF + EKF : Subsystem
  Heading Comparison : Scope  NumInputPorts=3
  Manual Switch1 : ManualSwitch
  Manual Switch2 : ManualSwitch  CurrentSetting=0
  Memory1 : Memory
  Mux1 : Mux  Inputs=2
  Mux3 : Mux  Inputs=2
  Selector : Selector  InputPortWidth=3  IndexOptions=Index vector (dialog)  Indices=1:2  OutputSizes=1
  Selector1 : Selector  InputPortWidth=3  IndexOptions=Index vector (dialog)  Indices=1:2  OutputSizes=1
  Selector2 : Selector  InputPortWidth=3  IndexOptions=Index vector (dialog)  Indices=3  OutputSizes=1
  Selector3 : Selector  InputPortWidth=3  IndexOptions=Index vector (dialog)  Indices=[1 2]  OutputSizes=1
  Selector4 : Selector  InputPortWidth=3  IndexOptions=Index vector (dialog)  Indices=3  OutputSizes=1
  Selector5 : Selector  InputPortWidth=3  IndexOptions=Index vector (dialog)  Indices=[1 2]  OutputSizes=1
  Selector6 : Selector  InputPortWidth=3  IndexOptions=Index vector (dialog)  Indices=3  OutputSizes=1
  Sensor Fusion - Complementary Filter : Subsystem
  Subsystem : Subsystem
  Subsystem1 : Subsystem
  Sum1 : Sum
  Terminator : Terminator
  Trigonometric Function : Trigonometry  Operator=cos
  Trigonometric Function1 : Trigonometry
  XY Plot : quarc_library/Sinks/Figures/XY Figure  figure_mode=Use figure window  figure_tag=figure1  axes_tag=axes1  plot_mode=Time-based  minimum_x=-2.5  maximum_x=2.5  minimum_y=-2  maximum_y=5  buffer_size=100  update_rate=1  initial_position="1    49  1920   982"  initial_visibility=off  sample_time=-1
      settings: SourceProductName=QUARC Targets
  bicycleModel : Subsystem
  get z_gyro : Selector  InputPortWidth=3  IndexOptions=Index vector (dialog)  Indices=[3]  OutputSizes=1
  xy signal maker : Subsystem
  currentPose [x,y,heading] (m,m,rad) : Outport
  wires:
  gyro [3] (rad/s)/1 -> get z_gyro/1
  get z_gyro/1 -> [z_gyro]
  Selector1/1 -> [xy]
  [steering] -> Memory1/1
  Demux/3 -> Gyro KF + EKF/5(th_gps)
  [speed] -> Gyro KF + EKF/1(speed)
  Demux/1 -> Gyro KF + EKF/3(x_gps)
  Gyro KF + EKF/1(Xhat) -> Selector4/1, Selector/1
  Memory1/1 -> Gyro KF + EKF/2(delta)
  [lidarPose] -> Demux/1
  Selector2/1 -> Subsystem1/1(Angle)
  Sensor Fusion - Complementary Filter/1(estimate) -> [senFusEstimate], Selector6/1  "pose"
  Fusion Comparison & Kalman Estimator/1(Kalman Pose) -> Selector2/1, Selector1/1
  [lidarPose] -> Sensor Fusion - Complementary Filter/3(correction)
  Subsystem/1(Mod_Angle) -> Heading Comparison/1, [heading]
  Selector/1 -> [Mitch_xy]
  [senFusEstimate] -> Fusion Comparison & Kalman Estimator/3(pose estimate)
  Selector6/1 -> Subsystem/1(Angle)
  [z_gyro] -> Gyro KF + EKF/6(thd_gyro)
  Subsystem1/1(Mod_Angle) -> Heading Comparison/3, [kal_heading]
  Selector4/1 -> Heading Comparison/2, [Mitch_heading]
  [poseRate] -> Fusion Comparison & Kalman Estimator/1(Pose dot)
  [lidarPose] -> Fusion Comparison & Kalman Estimator/2(pose)
  Demux/2 -> Gyro KF + EKF/4(y_gps)
  [speed] -> Sensor Fusion - Complementary Filter/1(car speed)
  Mux1/1 -> [currPose], currentPose [x,y,heading] (m,m,rad)/1
  Manual Switch1/1 -> Mux1/2
  [heading] -> Trigonometric Function1/1, Trigonometric Function/1
  Trigonometric Function/1 -> Mux3/1
  [heading] -> Manual Switch1/1
  [Mitch_xy] -> Manual Switch2/2
  Sum1/1 -> Mux1/1
  Trigonometric Function1/1 -> Mux3/2
  [xy] -> Manual Switch2/1
  [Mitch_heading] -> Manual Switch1/2
  Manual Switch2/1 -> Sum1/1
  Gain1/1 -> Sum1/2
  Mux3/1 -> Gain1/1
  carSpeed [1] (m/s)/1 -> [speed]
  steering [1] (rad)/1 -> [steering]
  newLidarReading [1] (bool)/1 -> [newLidarReading]
  lidarPose [x,y,heading] (m,m,rad)/1 -> [lidarPose]
  bicycleModel/1("poseRate (m/s, m/s, rad/s)") -> [poseRate]
  [poseRate] -> Sensor Fusion - Complementary Filter/2(rate)
  [kal_heading] -> bicycleModel/1(heading (rad))
  [newLidarReading] -> Gyro KF + EKF/7(newGPSData)
  Gyro KF + EKF/2(gyro_bias) -> Terminator/1
  [speed] -> bicycleModel/3(carSpeed (m/s))
  [steering] -> bicycleModel/2(steering [1] (rad))
  [z_gyro] -> bicycleModel/4(z_gyroscope (rad/s))
  [currPose] -> Selector5/1
  [lidarPose] -> Selector3/1
  xy signal maker/1(x) -> XY Plot/1
  xy signal maker/2(y) -> XY Plot/2
  Selector3/1 -> xy signal maker/1(xy 1)
  Selector5/1 -> xy signal maker/2(xy 2)

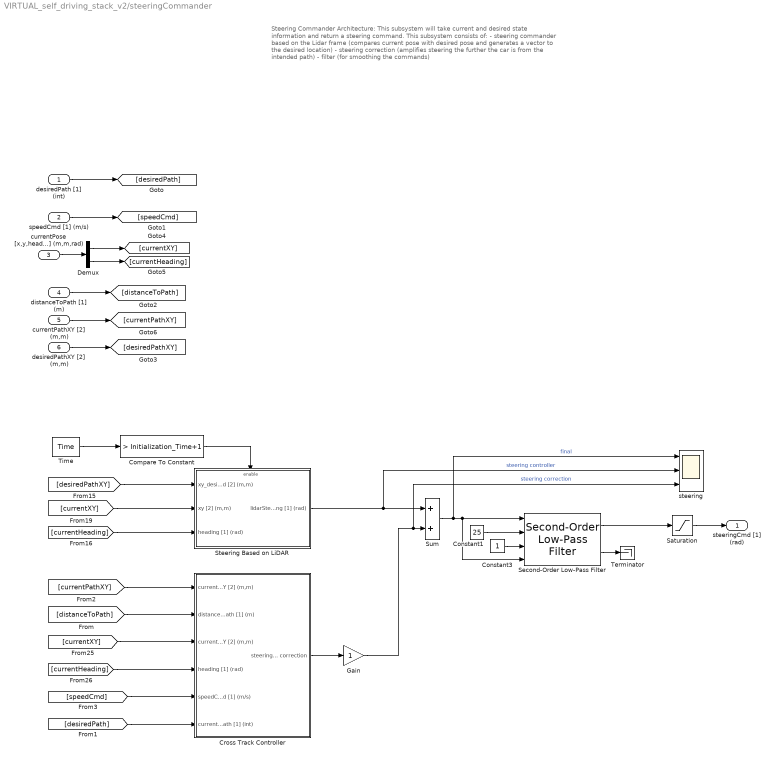
== system VIRTUAL_self_driving_stack_v2/steeringCommander ==
  note: Steering Commander Architecture:
      |
      | This subsystem will take current and desired state information and return a steering command.
      |
      | This subsystem consists of:
      |
      | - steering commander based on the Lidar frame (compares current pose with desired pose and generates a vector to the desired location)
      | - steering correction (amplifies steering the further the car is from the intended path)
      | - filter (for smoothing the commands)
  desiredPath [1] (int) : Inport
  speedCmd [1] (m/s) : Inport  Port=2
  currentPose [x,y,heading] (m,m,rad) : Inport  Port=3
  distanceToPath [1] (m) : Inport  Port=4
  currentPathXY [2] (m,m) : Inport  Port=5
  desiredPathXY [2] (m,m) : Inport  Port=6
  Compare To Constant : simulink/Logic and Bit Operations/Compare To Constant  relop=>  const=Initialization_Time+1  OutDataTypeStr=boolean
  Constant1 : Constant  Value=25
  Constant3 : Constant
  Cross Track Controller : Subsystem
  Demux : Demux  Outputs=2
  Gain : Gain
  Saturation : Saturate
  Second-Order Low-Pass Filter : quarc_library/Continuous/Second-Order Low-Pass Filter  params_source=External (input ports)  input_width=1  input_zeta=1  input_init=0
  Steering Based on LiDAR : Subsystem
  Sum : Sum
  Terminator : Terminator
  Time : quarc_library/Sources/Time/Time  time_source=Wall clock  sample_time=qc_get_step_size
  steering : Scope  NumInputPorts=3
  steeringCmd [1] (rad) : Outport
  wires:
  Demux/1 -> [currentXY]
  currentPose [x,y,heading] (m,m,rad)/1 -> Demux/1
  [desiredPathXY] -> Steering Based on LiDAR/1(xy_desired [2] (m,m))
  Steering Based on LiDAR/1(lidarSteering [1] (rad)) -> steering/2, Sum/1  "steering controller"
  [currentHeading] -> Cross Track Controller/4(heading [1] (rad))
  Demux/2 -> [currentHeading]
  [currentXY] -> Cross Track Controller/3(currentXY [2] (m,m))
  [currentXY] -> Steering Based on LiDAR/2(xy [2] (m,m))
  Cross Track Controller/1(steering correction) -> Gain/1
  desiredPath [1] (int)/1 -> [desiredPath]
  [desiredPath] -> Cross Track Controller/6(currentPath [1] (int))
  Sum/1 -> steering/1, Second-Order Low-Pass Filter/4, Second-Order Low-Pass Filter/1  "final"
  Constant3/1 -> Second-Order Low-Pass Filter/3
  Second-Order Low-Pass Filter/1 -> Saturation/1
  Second-Order Low-Pass Filter/2 -> Terminator/1
  Constant1/1 -> Second-Order Low-Pass Filter/2
  speedCmd [1] (m/s)/1 -> [speedCmd]
  [speedCmd] -> Cross Track Controller/5(speedCmd [1] (m/s))
  Time/1 -> Compare To Constant/1
  Compare To Constant/1 -> Steering Based on LiDAR/Enable
  distanceToPath [1] (m)/1 -> [distanceToPath]
  desiredPathXY [2] (m,m)/1 -> [desiredPathXY]
  currentPathXY [2] (m,m)/1 -> [currentPathXY]
  [distanceToPath] -> Cross Track Controller/2(distanceToPath [1] (m))
  [currentPathXY] -> Cross Track Controller/1(currentPathXY [2] (m,m))
  Saturation/1 -> steeringCmd [1] (rad)/1
  Gain/1 -> steering/3, Sum/2  "steering correction"
  [currentHeading] -> Steering Based on LiDAR/3(heading [1] (rad))

== system VIRTUAL_self_driving_stack_v2/writeToQCarDAC ==
  note: 11: LED left outside brake light
      | 12: LED left inside brake light
      | 12: LED right inside brake light
      | 13: LED right outside brake fight
      | 14: LED left reverse light
      | 15: LED right reverse light
      | 16: LED left rear signal
      | 17: LED right rear signal
      | 18: LED left outside headlight
      | 19: LED left middle headlight
      | 20: LED left inside headlight
      | 21: LED right inside headlight
      | 22: LED right middle headlight
      | 23: LED right outside headlight
      | 24: LED left front signal
      | 25: LED right front signal
  motor_cmd [1] (%) : Inport
  steering_cmd [1] (rad) : Inport  Port=2
  leds [14] (bool) : Inport  Port=3
  ledStrip [R,G,B] (%) : Inport  Port=4
  Gain : Gain
  HIL Write : quarc_library/Data Acquisition/Generic/Immediate I//O/HIL Write  object_name=HIL-2  analog_channels=[]  pwm_channels=[]  digital_channels=[11:26]  other_channels=[1000 11000]  sample_time=-1  active=on  vector_input=on
  LED Strip : quarc_library/Devices/Third-Party/Displays/LED Strip  led_type=AAAF5050-MC-K12  uri=tcpip://localhost:18969  mode=uniform  max_leds=33  initial_red=[0.000]  initial_green=[1.000]  initial_blue=[0.000]  final_red=[0]  final_green=[0]  final_blue=[0]  sample_time=ImageDisplay_Sample_Time  use_vectors=off  active=off
      settings: SourceProductName=QUARC Targets
  Mux : Mux  Inputs=2
  Steering Bias : Bias  Bias=-0.05  SaturateOnIntegerOverflow=off
  Terminator : Terminator
  motor sat : Saturate  UpperLimit=.6  LowerLimit=-0.6
  steering sat : Saturate
  wires:
  ledStrip [R,G,B] (%)/1 -> LED Strip/1
  steering_cmd [1] (rad)/1 -> Steering Bias/1
  motor sat/1 -> Mux/2
  steering sat/1 -> Mux/1
  leds [14] (bool)/1 -> HIL Write/1
  Steering Bias/1 -> Gain/1
  motor_cmd [1] (%)/1 -> motor sat/1
  LED Strip/1 -> Terminator/1
  Gain/1 -> steering sat/1
  Mux/1 -> HIL Write/2

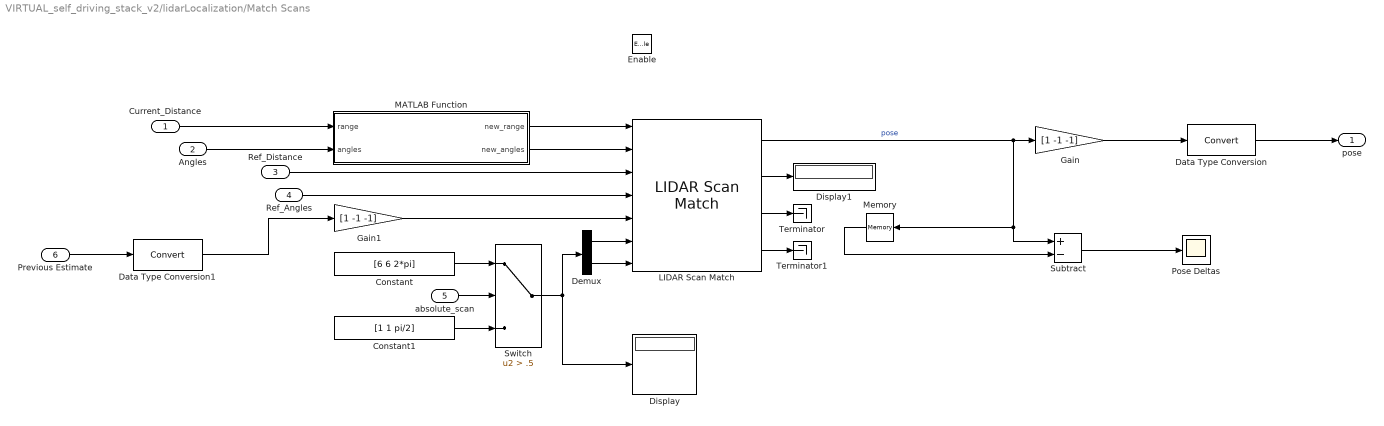
== system VIRTUAL_self_driving_stack_v2/lidarLocalization/Match Scans ==
  Current_Distance : Inport
  Angles : Inport  Port=2
  Ref_Distance : Inport  Port=3
  Ref_Angles : Inport  Port=4
  absolute_scan : Inport  Port=5
  Previous Estimate : Inport  Port=6
  Enable : EnablePort  PropagateVarSize=During execution
  Constant : Constant  Value=[6 6 2*pi]
  Constant1 : Constant  Value=[1 1 pi/2]
  Data Type Conversion : DataTypeConversion  SaturateOnIntegerOverflow=off  RndMeth=Floor
  Data Type Conversion1 : DataTypeConversion  SaturateOnIntegerOverflow=off  RndMeth=Floor
  Demux : Demux  Outputs=2
  Display : Display
  Display1 : Display
  Gain : Gain  Gain=[1 -1 -1]
  Gain1 : Gain  Gain=[1 -1 -1]
  LIDAR Scan Match : quarc_library/Image Processing/Generic/LIDAR Scan Match  mode=Variable-size input  resolution=35  max_range=8  use_initial_pose=on
      settings: SourceProductName=QUARC Targets
  MATLAB Function : MATLAB Function  TreatAsAtomicUnit=on
  Memory : Memory  InitialCondition=[0 0 0]  InheritSampleTime=on  LinearizeMemory=on  LinearizeAsDelay=on
  Pose Deltas : Scope
  Subtract : Sum  Inputs=+-
  Switch : Switch  Criteria=u2 > Threshold  Threshold=.5  SaturateOnIntegerOverflow=off  InputSameDT=off
  Terminator : Terminator
  Terminator1 : Terminator
  pose : Outport
  wires:
  LIDAR Scan Match/1 -> Subtract/1, Memory/1, Gain/1  "pose"
  Ref_Distance/1 -> LIDAR Scan Match/3
  Ref_Angles/1 -> LIDAR Scan Match/4
  Gain/1 -> Data Type Conversion/1
  Memory/1 -> Subtract/2
  absolute_scan/1 -> Switch/2
  Switch/1 -> Demux/1, Display/1
  Demux/1 -> LIDAR Scan Match/6
  Demux/2 -> LIDAR Scan Match/7
  Constant/1 -> Switch/1
  Constant1/1 -> Switch/3
  Data Type Conversion/1 -> pose/1
  MATLAB Function/1(new_range) -> LIDAR Scan Match/1
  MATLAB Function/2(new_angles) -> LIDAR Scan Match/2
  Subtract/1 -> Pose Deltas/1
  Previous Estimate/1 -> Data Type Conversion1/1
  Gain1/1 -> LIDAR Scan Match/5
  Data Type Conversion1/1 -> Gain1/1
  Current_Distance/1 -> MATLAB Function/1(range)
  Angles/1 -> MATLAB Function/2(angles)
  LIDAR Scan Match/3 -> Terminator/1
  LIDAR Scan Match/4 -> Terminator1/1
  LIDAR Scan Match/2 -> Display1/1

== system VIRTUAL_self_driving_stack_v2/lidarLocalization/RisingEdge ==
  Input : Inport
  Logical Operator1 : Logic  AllPortsSameDT=off
  Logical Operator2 : Logic  Operator=NOT  AllPortsSameDT=off
  Memory : Memory  InheritSampleTime=on  LinearizeMemory=on
  RisingEdgeTrigger : Outport  VectorParamsAs1DForOutWhenUnconnected=off
  wires:
  Logical Operator1/1 -> RisingEdgeTrigger/1
  Logical Operator2/1 -> Logical Operator1/2
  Memory/1 -> Logical Operator2/1
  Input/1 -> Logical Operator1/1, Memory/1

== system VIRTUAL_self_driving_stack_v2/lidarLocalization/rising edge latch ==
  rising edge trigger : Inport
  input : Inport  Port=2
  untriggered output : Inport  Port=3
  Latch Input : Subsystem  TreatAsAtomicUnit=on
  Switch : Switch  Threshold=0.5  SaturateOnIntegerOverflow=off  InputSameDT=off
  output : Outport  VectorParamsAs1DForOutWhenUnconnected=off
  wires:
  untriggered output/1 -> Switch/3
  Switch/1 -> output/1
  Latch Input/1(Latch) -> Switch/1
  Latch Input/2(Executed) -> Switch/2
  input/1 -> Latch Input/1(Input)
  rising edge trigger/1 -> Latch Input/Trigger
